simulink model "PD"  (R2016a)
settings: Solver=VariableStepAuto  StartTime=0.0  StopTime=10.0  RelTol=1e-3
undefined symbols (not defined in the file or in its folder): invMbarra, kd_pd, kp_pd
libraries: simulink_extras x6
settings Model: Creator=gabri  LastModifiedBy=gabri
settings GRTTargetCC: GeneratePreprocessorConditionals=Use local settings

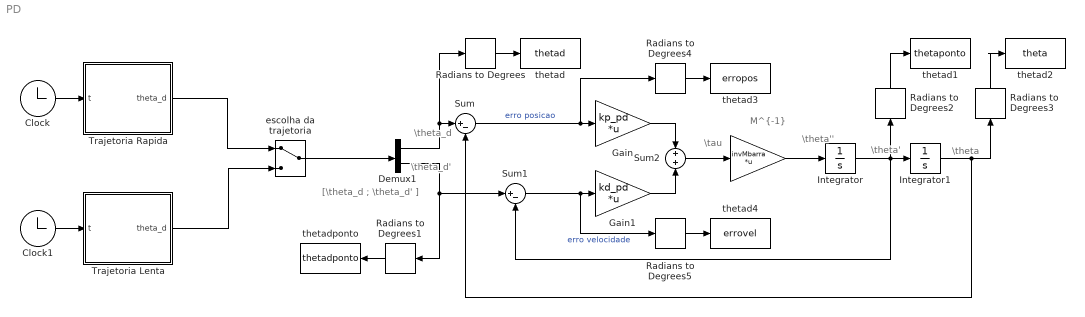
== system PD ==
  note: \theta''
  note: M^{-1}
  note: \tau
  note: \theta_d
  note: [\theta_d ; \theta_d' ]
  note: \theta_d'
  note: \theta'
  note: \theta
  "   " : Gain  Gain=invMbarra  Multiplication=Matrix(K*u)
  Clock : Clock
  Clock1 : Clock
  Demux1 : Demux  Outputs=2
  Gain : Gain  Gain=kp_pd  Multiplication=Matrix(K*u)
  Gain1 : Gain  Gain=kd_pd  Multiplication=Matrix(K*u)
  Integrator : Integrator
  Integrator1 : Integrator  InitialCondition=[-pi/2;pi]
  Radians to Degrees{,1..5} (6 alike) : simulink_extras/Transformations/Radians to Degrees
  Sum : Sum  Inputs=|+-
  Sum1 : Sum  Inputs=|+-
  Sum2 : Sum  Inputs=+|+
  Trajetoria Lenta : MATLAB Function  TreatAsAtomicUnit=on
  Trajetoria Rapida : MATLAB Function  TreatAsAtomicUnit=on
  "escolha da trajetoria " : ManualSwitch
  thetad : ToWorkspace  VariableName=thetad  SaveFormat=Timeseries  SampleTime=-1
  thetad1 : ToWorkspace  VariableName=thetaponto  SaveFormat=Timeseries  SampleTime=-1
  thetad2 : ToWorkspace  VariableName=theta  SaveFormat=Timeseries  SampleTime=-1
  thetad3 : ToWorkspace  VariableName=erropos  SaveFormat=Timeseries  SampleTime=-1
  thetad4 : ToWorkspace  VariableName=errovel  SaveFormat=Timeseries  SampleTime=-1
  thetadponto : ToWorkspace  VariableName=thetadponto  SaveFormat=Timeseries  SampleTime=-1
  wires:
  Clock/1 -> Trajetoria Rapida/1(t)
  Clock1/1 -> Trajetoria Lenta/1(t)
  Trajetoria Lenta/1(theta_d) -> "escolha da trajetoria "/2
  "escolha da trajetoria "/1 -> Demux1/1
  Trajetoria Rapida/1(theta_d) -> "escolha da trajetoria "/1
  Demux1/1 -> Sum/1, Radians to Degrees/1
  Sum/1 -> Radians to Degrees4/1, Gain/1  "erro posicao"
  Demux1/2 -> Sum1/1, Radians to Degrees1/1
  Sum1/1 -> Radians to Degrees5/1, Gain1/1  "erro velocidade"
  Gain/1 -> Sum2/1
  Gain1/1 -> Sum2/2
  Sum2/1 -> "   "/1
  "   "/1 -> Integrator/1
  Integrator/1 -> Sum1/2, Radians to Degrees2/1, Integrator1/1
  Integrator1/1 -> Radians to Degrees3/1, Sum/2
  Radians to Degrees/1 -> thetad/1
  Radians to Degrees1/1 -> thetadponto/1
  Radians to Degrees2/1 -> thetad1/1
  Radians to Degrees3/1 -> thetad2/1
  Radians to Degrees4/1 -> thetad3/1
  Radians to Degrees5/1 -> thetad4/1

== matlab function PD/Trajetoria Lenta ==
  data: theta_d output; t input
function theta_d = fcn(t)
theta_d_l = [(-0.75*cos(pi*t/2))-0.75; (-0.75*cos(pi*t/2))+3.75];

thetadot_d_l = [0.75*(pi/2)*sin(pi*t/2); 0.75*(pi/2)*sin(pi*t/2)];

theta_d = [theta_d_l;thetadot_d_l];

== matlab function PD/Trajetoria Rapida ==
  data: theta_d output; t input
function theta_d = fcn(t)
theta_d_r = [(-0.75*cos(pi*t))-0.75; (-0.75*cos(pi*t))+3.75];

thetadot_d_r = [0.75*pi*sin(pi*t); 0.75*pi*sin(pi*t)];

theta_d = [theta_d_r; thetadot_d_r];
